simulink model "modbusmaster_exec"  (Simulink 3.00)
libraries: execlib x6

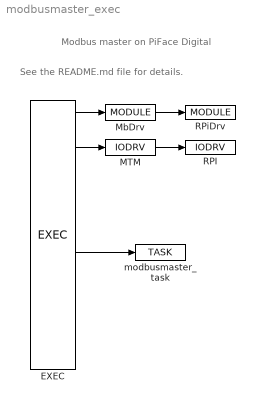
== system modbusmaster_exec ==
  note: See the README.md file for details.
  note: Modbus master on PiFace Digital
  EXEC : execlib/EXEC  target=Generic target device  tick=0.05  ntick0=2  ntick1=50  ntick2=100  ntick3=1200  pri0=5  pri1=9  pri2=13  pri3=18
  MTM : execlib/IODRV  module=MbDrv  classname=MtmDrv  cfgname=modbusmaster_iocfg.rio  factor=10  stack=10240  pri=3  timer=off
  MbDrv : execlib/MODULE
  RPI : execlib/IODRV  module=RPiDrv  classname=RPiDrv  factor=1  stack=10240  pri=3  timer=off
  RPiDrv : execlib/MODULE
  modbusmaster_task : execlib/TASK  factor=1  start=0  stop=1  stack=10240  MDLOPEN=on
  wires:
  EXEC/1 -> MbDrv/1
  EXEC/2 -> MTM/1
  EXEC/5 -> modbusmaster_task/1
  MTM/1 -> RPI/1
  MbDrv/1 -> RPiDrv/1
